simulink model "VMC_DSPLib_Solution_Stage3"  (R2025a)
settings: Solver=VariableStepAuto  StartTime=0.0  StopTime=5000  RelTol=1e-3
PreLoadFcn:
  | CreateFilter;
InitFcn:
  | CreateFilter;
undefined symbols (not defined in the file or in its folder): cfi, hb1, hb2, hb3, i, L, None, Shift1, Shift2, Shift3, ShiftCF, vsva2197, xcvc1902
libraries: aieDSP x4, dspmlti4 x3, aieBasic x1, dspsrcs4 x1, aieUtilities x1, vmcUtilities x1
settings Model: Creator=robg  LastModifiedBy=robg
settings ModelReferenceCC: EnableRefExpFcnMdlSchedulingChecks=on
settings RTWCC: GPUComputeCapability=3.5

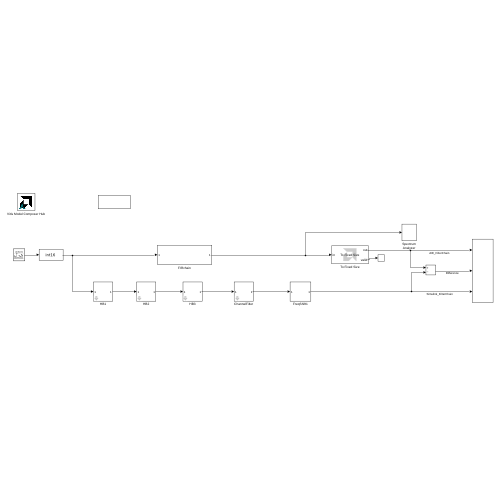
[thumbnail: Simulink's stored preview of the top-level diagram]
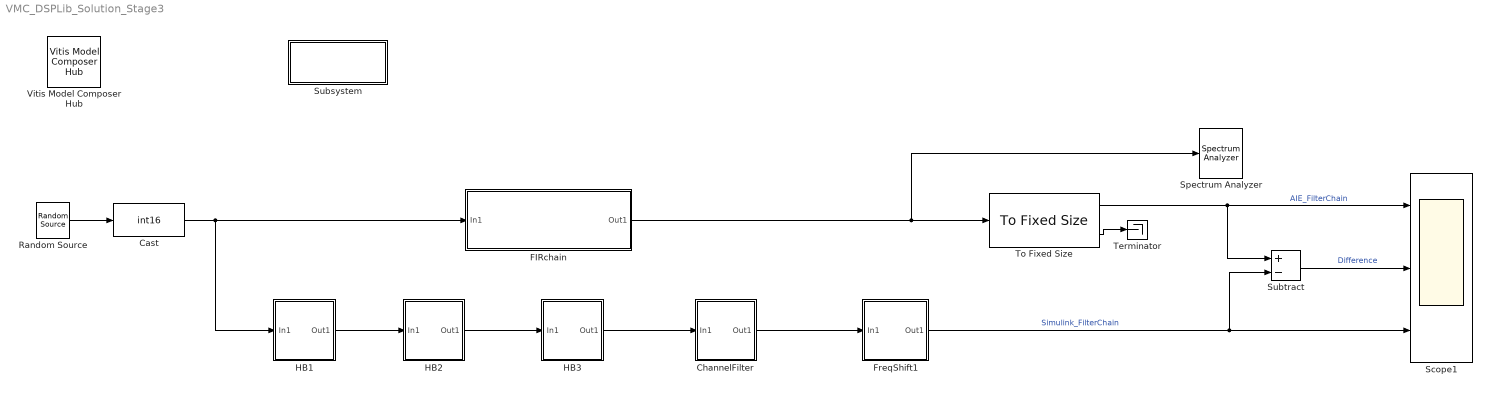
== system VMC_DSPLib_Solution_Stage3 ==
  Cast : DataTypeConversion  OutDataTypeStr=int16  SaturateOnIntegerOverflow=off  RndMeth=Floor
  ChannelFilter : Subsystem  mask{COEFFS=cfi, Shift=ShiftCF}
      mask prompts: COEFFS "Coefficients"; Shift "Final Shift"
  FIRchain : Subsystem
  FreqShift1 : Subsystem
  HB1 : Subsystem  mask{COEFFS=hb1, Shift=Shift1}
      mask prompts: COEFFS "Coefficients"; Shift "Final Shift"
  HB2 : Subsystem  mask{COEFFS=hb2, Shift=Shift2}
      mask prompts: COEFFS "Coefficients"; Shift "Final Shift"
  HB3 : Subsystem  mask{COEFFS=hb3, Shift=Shift3}
      mask prompts: COEFFS "Coefficients"; Shift "Final Shift"
  Random Source : dspsrcs4/Random Source  SrcType=Uniform  MinVal=-20000  MaxVal=20000  MeanVal=0  VarVal=1  RepMode=Specify seed  rawSeed=1  IsInherit=off  SampTime=1  SampFrame=2048  OutComplex=Complex  DataType=double  SimulateUsing=Interpreted execution
  Scope1 : Scope  NumInputPorts=3
      settings: ActiveDisplayYMinimum=-19139.5  ActiveDisplayYMaximum=19715.5
  Spectrum Analyzer : SpectrumAnalyzer  WindowPosition=[560.000000,350.000000,800.000000,500.000000,]  Visible=on  ScopeFrameLocation=window  SampleRate=0.125  Span=0.125  StartFrequency=-0.0625  StopFrequency=0.0625  AveragingMethod=Exponential  YLimits=[19.3644 90.7876]  AllowFFTLengthLessThanSamplesPerUpdate=on  DefaultConfigurationName=spbscopes.SpectrumAnalyzerBlockCfg  IsFrequencyInputMode=0  FrequencyVectorPort=0  FrequencyVectorFromPort=0  FrequencyInputRBWPort=0  FrequencyInputRBWFromPort=0
  Subsystem : Subsystem
      settings: OpenFcn=open('CreateFilter.m');
  Subtract : Sum  Inputs=+-
  Terminator : Terminator
  To Fixed Size : aieUtilities/To Fixed Size  Mode=Produce a valid output signal  OutputSize=256  CopyMethod=Buffer samples to form output  HasStatusOutput=on
  Vitis Model Composer Hub : vmcUtilities/Vitis Model Composer Hub  Tag=genX  CodeGeneration=off  SubsystemName=FIRchain  BlockHierPath=VMC_DSPLib_Solution_Stage3/FIRchain  SubsystemType=AIENode  StartColumn=1  NumberOfColumns=1  TargetDirectory=./code  exportDesign=off  analyzeDesign=on  validateDesignOnHw=off  ExportType=AI Engines  IpVendor=xilinx.com  IpLibrary=hls  IpVersion=1.0  IpHWLanguage=Verilog  AieCompilerOptions={}  AieSimulatorOptions={}  CreateTestbench=on  TestbenchStackSize=10  RunRtlSim=off  RunCSim=off  RunAieSim=on  enableSimulationTimeout=on  enableGraphIterations=on  AieSimTimeout=50000  AieGraphIterations=-1  RunAieSimProfiling=on  LaunchVitisAnalyzer=on  PlotOutput=off  RunX86Sim=off  X86SimTimeout=10  GenHwImage=off  GenLibadfXo=off  GenHwValidationCode=off  PlatformType=Not Specified  HwSystemType=Baremetal  HwValidationTarget=hw  ProjDevice=xcvc1902-vsva2197-1LHP-i-L  ProjDevicePart=xcvc1902-vsva2197-1LHP-i-L  AIEType=AIE  SamplePeriod=-1  ClockFrequency=200  DataPathParallelism=1  xilinxfamily=versalaicore  part=xcvc1902  speed=-1LHP-i-L  package=vsva2197  directory=./code  testbench=off  incr_netlist=off  synthesis_tool=Vivado  clock_wrapper=Clock Enables  dbl_ovrd=According to Block Masks  dcm_input_clock_period=10  sysclk_period=10  simulink_period=1  eval_field=0  IPInfoJsonString="{\"DUTSubsystemName\":\"FIRchain\",\"AIESubsystem\":{\"SubsystemName\":\"FIRchain\",\"TargetDirectory\":\"./code\",\"AIEArrayConfig\":\"Use entire AIE array\",\"StartColumn\":\"0\",\"NumberOfColumns\":\"1\"},\"SubsystemTag\":\"AIENode\"}"  LogFileName=/group/xcoswmktg2/robg/git/Vitis-Tutorials/Internal-Fork/AI_Engine_Development/AIE/Feature_Tutorials/10-aie-dsp-lib-model-composer/code/model_composer.log  NThreads=4  IPConfigFile=/tmp/vmctmp-2277828951318312850/VMC_DSPLib_Solution_Stage3_ipconfig.json
  wires:
  Random Source/1 -> Cast/1
  Cast/1 -> FIRchain/1(In1), HB1/1(In1)
  To Fixed Size/2 -> Terminator/1
  HB1/1(Out1) -> HB2/1(In1)
  To Fixed Size/1 -> Scope1/1, Subtract/1  "AIE_FilterChain"
  Subtract/1 -> Scope1/2  "Difference"
  HB2/1(Out1) -> HB3/1(In1)
  HB3/1(Out1) -> ChannelFilter/1(In1)
  ChannelFilter/1(Out1) -> FreqShift1/1(In1)
  FreqShift1/1(Out1) -> Scope1/3, Subtract/2  "Simulink_FilterChain"
  FIRchain/1(Out1) -> To Fixed Size/1, Spectrum Analyzer/1

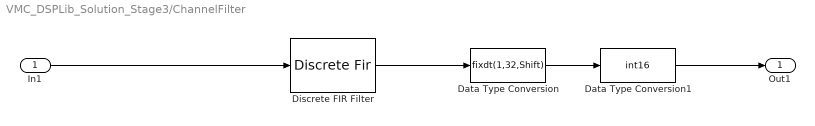
== system VMC_DSPLib_Solution_Stage3/ChannelFilter ==
  In1 : Inport
  Data Type Conversion : DataTypeConversion  OutDataTypeStr=fixdt(1,32,Shift)  ConvertRealWorld=Stored Integer (SI)  SaturateOnIntegerOverflow=off  RndMeth=Floor
  Data Type Conversion1 : DataTypeConversion  OutDataTypeStr=int16  RndMeth=Floor
  Discrete FIR Filter : DiscreteFir  Coefficients=COEFFS  InputProcessing=Columns as channels (frame based)
  Out1 : Outport
  wires:
  Data Type Conversion/1 -> Data Type Conversion1/1
  In1/1 -> Discrete FIR Filter/1
  Discrete FIR Filter/1 -> Data Type Conversion/1
  Data Type Conversion1/1 -> Out1/1

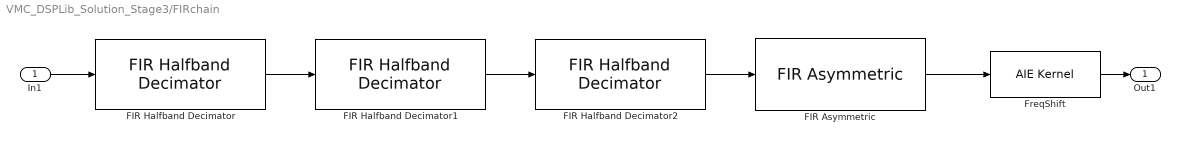
== system VMC_DSPLib_Solution_Stage3/FIRchain ==
  In1 : Inport
  FIR Asymmetric : aieDSP/FIR Asymmetric  data_type=cint16  coef_type=int16  use_coeff_reload=off  num_outputs=off  coeff=cfi  fir_length=32  input_window_size=256  shift_val=ShiftCF  rnd_mode=Floor  sat_mode=0-None  casc_length=1  AIE_VARIANT=1  TP_API=0  dual_ip=0  ssr=1  blockJsonConstraints=[]  blockJsonConstraintsInternal=[]  spec=vmc_fir_sr_asym.json  SerializedMaskParamNames=[]  SerializedMaskParamValues=[]  SerializedMaskParamVisibilities=[]  block_type=FIR Asymmetric  SerializedMaskParamDataypes=typename|typename|uint|uint|coef_type|uint|uint|uint|uint|uint|uint|uint|uint|uint|uint  SerializedMaskParamEnumStrArr=0|0|0|0|0|0|0|0|Floor,Ceiling,Round to positive infinity,Round to negative infinity,Round symmetrical to infinity,Round symmetrical to zero,Round convergent to even,Round convergent to odd|0-None,1-Asymmetric,3-Symmetric|0|0|0|0|0  SerializedMaskParamEnumValArr=0|0|0|0|0|0|0|0|0,1,2,3,4,5,6,7|0,1,3|0|0|0|0|0  SerializedMaskParamVectorArr=0|0|0|0|1|0|0|0|0|0|0|0|0|0|0  SerializedMaskParamKeys=TT_DATA|TT_COEFF|TP_USE_COEFF_RELOAD|TP_NUM_OUTPUTS|coeff|TP_FIR_LEN|TP_INPUT_WINDOW_VSIZE|TP_SHIFT|TP_RND|TP_SAT|TP_CASC_LEN|AIE_VARIANT|TP_API|TP_DUAL_IP|TP_SSR
  FIR Halfband Decimator : aieDSP/FIR Halfband Decimator  data_type=cint16  coef_type=int16  use_coeff_reload=off  dual_ip=off  num_outputs=off  coeff=hb1_aie  fir_length=31  input_window_size=2048  shift_val=Shift1  rnd_mode=Floor  sat_mode=0-None  deci_poly=1  casc_length=2  AIE_VARIANT=1  TP_API=0  ssr=1  blockJsonConstraints=[]  blockJsonConstraintsInternal=[]  spec=vmc_fir_decimate_hb.json  SerializedMaskParamNames=[]  SerializedMaskParamValues=[]  SerializedMaskParamVisibilities=[]  block_type=FIR Halfband Decimator  SerializedMaskParamDataypes=typename|typename|uint|uint|uint|coef_type|uint|uint|uint|uint|uint|uint|uint|uint|uint|uint  SerializedMaskParamEnumStrArr=0|0|0|0|0|0|0|0|0|Floor,Ceiling,Round to positive infinity,Round to negative infinity,Round symmetrical to infinity,Round symmetrical to zero,Round convergent to even,Round convergent to odd|0-None,1-Asymmetric,3-Symmetric|0|0|0|0|0  SerializedMaskParamEnumValArr=0|0|0|0|0|0|0|0|0|0,1,2,3,4,5,6,7|0,1,3|0|0|0|0|0  SerializedMaskParamVectorArr=0|0|0|0|0|1|0|0|0|0|0|0|0|0|0|0  SerializedMaskParamKeys=TT_DATA|TT_COEFF|TP_USE_COEFF_RELOAD|TP_DUAL_IP|TP_NUM_OUTPUTS|coeff|TP_FIR_LEN|TP_INPUT_WINDOW_VSIZE|TP_SHIFT|TP_RND|TP_SAT|TP_PARA_DECI_POLY|TP_CASC_LEN|AIE_VARIANT|TP_API|TP_SSR
  FIR Halfband Decimator1 : aieDSP/FIR Halfband Decimator  data_type=cint16  coef_type=int16  use_coeff_reload=off  dual_ip=off  num_outputs=off  coeff=hb2_aie  fir_length=31  input_window_size=1024  shift_val=Shift2  rnd_mode=Floor  sat_mode=0-None  deci_poly=1  casc_length=2  AIE_VARIANT=1  TP_API=0  ssr=1  blockJsonConstraints=[]  blockJsonConstraintsInternal=[]  spec=vmc_fir_decimate_hb.json  SerializedMaskParamNames=[]  SerializedMaskParamValues=[]  SerializedMaskParamVisibilities=[]  block_type=FIR Halfband Decimator  SerializedMaskParamDataypes=typename|typename|uint|uint|uint|coef_type|uint|uint|uint|uint|uint|uint|uint|uint|uint|uint  SerializedMaskParamEnumStrArr=0|0|0|0|0|0|0|0|0|Floor,Ceiling,Round to positive infinity,Round to negative infinity,Round symmetrical to infinity,Round symmetrical to zero,Round convergent to even,Round convergent to odd|0-None,1-Asymmetric,3-Symmetric|0|0|0|0|0  SerializedMaskParamEnumValArr=0|0|0|0|0|0|0|0|0|0,1,2,3,4,5,6,7|0,1,3|0|0|0|0|0  SerializedMaskParamVectorArr=0|0|0|0|0|1|0|0|0|0|0|0|0|0|0|0  SerializedMaskParamKeys=TT_DATA|TT_COEFF|TP_USE_COEFF_RELOAD|TP_DUAL_IP|TP_NUM_OUTPUTS|coeff|TP_FIR_LEN|TP_INPUT_WINDOW_VSIZE|TP_SHIFT|TP_RND|TP_SAT|TP_PARA_DECI_POLY|TP_CASC_LEN|AIE_VARIANT|TP_API|TP_SSR
  FIR Halfband Decimator2 : aieDSP/FIR Halfband Decimator  data_type=cint16  coef_type=int16  use_coeff_reload=off  dual_ip=off  num_outputs=off  coeff=hb3_aie  fir_length=31  input_window_size=512  shift_val=Shift3  rnd_mode=Floor  sat_mode=0-None  deci_poly=1  casc_length=2  AIE_VARIANT=1  TP_API=0  ssr=1  blockJsonConstraints=[]  blockJsonConstraintsInternal=[]  spec=vmc_fir_decimate_hb.json  SerializedMaskParamNames=[]  SerializedMaskParamValues=[]  SerializedMaskParamVisibilities=[]  block_type=FIR Halfband Decimator  SerializedMaskParamDataypes=typename|typename|uint|uint|uint|coef_type|uint|uint|uint|uint|uint|uint|uint|uint|uint|uint  SerializedMaskParamEnumStrArr=0|0|0|0|0|0|0|0|0|Floor,Ceiling,Round to positive infinity,Round to negative infinity,Round symmetrical to infinity,Round symmetrical to zero,Round convergent to even,Round convergent to odd|0-None,1-Asymmetric,3-Symmetric|0|0|0|0|0  SerializedMaskParamEnumValArr=0|0|0|0|0|0|0|0|0|0,1,2,3,4,5,6,7|0,1,3|0|0|0|0|0  SerializedMaskParamVectorArr=0|0|0|0|0|1|0|0|0|0|0|0|0|0|0|0  SerializedMaskParamKeys=TT_DATA|TT_COEFF|TP_USE_COEFF_RELOAD|TP_DUAL_IP|TP_NUM_OUTPUTS|coeff|TP_FIR_LEN|TP_INPUT_WINDOW_VSIZE|TP_SHIFT|TP_RND|TP_SAT|TP_PARA_DECI_POLY|TP_CASC_LEN|AIE_VARIANT|TP_API|TP_SSR
  FreqShift : aieBasic/AIE Kernel  KernelAllAttrs=|  PortNames={'in'; 'out'}  PortSerializedTypes={'{Q2{R{Tadf::input_buffer{1{t{Scint16}}}}}}'; '{Q2{R{Tadf::output_buffer{1{t{Scint16}}}}}}'}  PortWindowSizes={2.560000000000000000e+02, 2.560000000000000000e+02}  PortWindowMargins={0.000000000000000000e+00, 0.000000000000000000e+00}  PortSynchronicities={'sync', 'sync'}  PortSignalSizes={0.000000000000000000e+00; 0.000000000000000000e+00}  FunctionTemplateSpecKind=implicit  FunctionTemplateParamNames={'FRAME_LENGTH'}  FunctionTemplateParamKinds={'nontype'}  FunctionTemplateParamTypes={'int'}  FunctionTemplateParamValues={'256'}  FunctionIndex=1  FunctionTabVisible=on  FunctionTemplateParamsVisible=on  FunctionDeclTypeOptions=|  FunctionDecl=|  FunctionTemplateParams={ 'FRAME_LENGTH', 'int', '256' }  FunctionTemplateParamsEnables={'off', 'off', 'on'}  PortAttrs={ 'input', 'in', 'adf::input_buffer< cint16 > & restrict', '256', '0', 'sync', ''; 'output', 'out', 'adf::output_buffer< cint16 > & restrict', '256', '', 'sync', '' }  PortAttrsEnables={'off', 'off', 'off', 'on', 'off', 'off', 'off';'off', 'off', 'off', 'on', 'off', 'off', 'off'}  SampleTime=-1  KernelHeaderFile=aiecode_src/FreqShift.h  KernelFunction=FreqShift  KernelSourceFile=aiecode_src/FreqShift.cpp  KernelSearchPaths={}  PreProcOptions={}  blockJsonConstraints=[]
      KernelAllAttrs=|
      | s[12;12;9;9;19;14;21;23;21;23;24;21;15;17;12;24;26;26;26;27;28;9;21;23;23;23;24;25;14;19;19;29]@FunctionNameDeclFileNamePortNamesPortTypesPortSerializedTypesPortDirectionsPortWindowSizeEnablesPortWindowMarginEnablesPortBufferSizeEnablesPortBufferMarginEnablesPortSynchronicityEnablesPortSignalSizeEnablesPortBufferSizesPortBufferMarginsFunctionDeclFunctionTemplateSpecKindFunctionTemplateParamNamesFunctionTemplateParamKindsFunctionTemplateParamTypesFunctionTemplateParamValuesFunctionTemplateParamEnablesClassDeclClassTemplateSpecKindClassTemplateParamNamesClassTemplateParamKindsClassTemplateParamTypesClassTemplateParamValuesClassTemplateParamEnablesClassCtorDeclsClassCtorParamNamesClassCtorParamTypesClassCtorParamSerializedTypes[1 1]@C[32 1]@t9@FreqShiftt29@../../aiecode_src/FreqShift.hC[2 1]@t2@int3@outC[2 1]@t38@adf::input_buffer< cint16 > & restrictt39@adf::output_buffer< cint16 > & restrictC[2 1]@t42@{Q2{R{Tadf::input_buffer{1{t{Scint16}}}}}}t43@{Q2{R{Tadf::output_buffer{1{t{Scint16}}}}}}C[2 1]@t5@inputt6@outputC[2 1]@l1@l1@C[2 1]@l1@l0@C[2 1]@l1@l1@C[2 1]@l0@l0@C[2 1]@l1@l1@C[2 1]@l0@l0@C[2 1]@nnC[2 1]@nnt133@template < int FRAME_LENGTH > 
      | void FreqShift(adf::input_buffer< cint16 > & restrict in, adf::output_buffer< cint16 > & restrict out)t8@implicitC[1 1]@t12@FRAME_LENGTHC[1 1]@t7@nontypeC[1 1]@t3@intC[1 1]@nC[1 1]@l1@nne[0 1]@e[0 1]@e[0 1]@e[0 1]@e[0 1]@e[0 1]@e[0 1]@e[0 1]@e[0 1]@
      FunctionDeclTypeOptions=|
      | C[1 1]@t135@template < int FRAME_LENGTH > 
      | void FreqShift(adf::input_buffer< cint16 > && restrict in, adf::output_buffer< cint16 > && restrict out)
      FunctionDecl=|
      | template < int FRAME_LENGTH > 
      | void FreqShift(adf::input_buffer< cint16 > && restrict in, adf::output_buffer< cint16 > && restrict out)
  Out1 : Outport
  wires:
  FIR Halfband Decimator2/1 -> FIR Asymmetric/1
  FIR Halfband Decimator/1 -> FIR Halfband Decimator1/1
  FIR Halfband Decimator1/1 -> FIR Halfband Decimator2/1
  FIR Asymmetric/1 -> FreqShift/1
  FreqShift/1 -> Out1/1
  In1/1 -> FIR Halfband Decimator/1

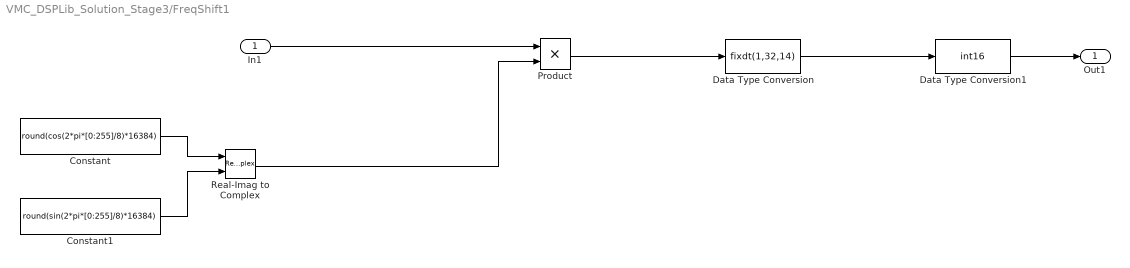
== system VMC_DSPLib_Solution_Stage3/FreqShift1 ==
  In1 : Inport
  Constant : Constant  Value=round(cos(2*pi*[0:255]/8)*16384)  SampleTime=2048
  Constant1 : Constant  Value=round(sin(2*pi*[0:255]/8)*16384)  SampleTime=2048
  Data Type Conversion : DataTypeConversion  OutDataTypeStr=fixdt(1,32,14)  ConvertRealWorld=Stored Integer (SI)  SaturateOnIntegerOverflow=off  RndMeth=Floor
  Data Type Conversion1 : DataTypeConversion  OutDataTypeStr=int16  RndMeth=Floor
  Product : Product
  Real-Imag to Complex : RealImagToComplex
  Out1 : Outport
  wires:
  In1/1 -> Product/1
  Product/1 -> Data Type Conversion/1
  Real-Imag to Complex/1 -> Product/2
  Data Type Conversion1/1 -> Out1/1
  Constant/1 -> Real-Imag to Complex/1
  Constant1/1 -> Real-Imag to Complex/2
  Data Type Conversion/1 -> Data Type Conversion1/1

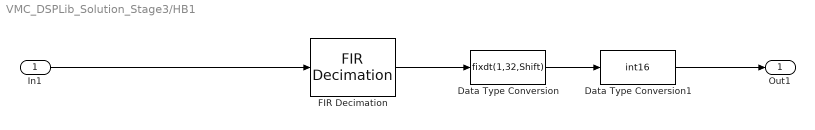
== system VMC_DSPLib_Solution_Stage3/HB1 ==
  In1 : Inport
  Data Type Conversion : DataTypeConversion  OutDataTypeStr=fixdt(1,32,Shift)  ConvertRealWorld=Stored Integer (SI)  SaturateOnIntegerOverflow=off  RndMeth=Floor
  Data Type Conversion1 : DataTypeConversion  OutDataTypeStr=int16  RndMeth=Floor
  FIR Decimation : dspmlti4/FIR Decimation  FilterSource=Dialog parameters  h=COEFFS  D=2  filtStruct=Direct form  FilterObject=FDECIM  InputProcessing=Columns as channels (frame based)  framing=Enforce single-rate processing  AllowArbitraryInputLength=off  inputOffset=0  outputBufInitCond=0  roundingMode=Floor  overflowMode=off  firstCoeffDataTypeStr=Inherit: Same word length as input  firstCoeffMin=[]  firstCoeffMax=[]  firstCoeffLastDataTypeStr=Inherit: Same word length as input  outputDataTypeStr=Inherit: Same as accumulator  outputMin=[]  outputMax=[]  outputLastDataTypeStr=Inherit: Same as accumulator
  Out1 : Outport
  wires:
  Data Type Conversion1/1 -> Out1/1
  FIR Decimation/1 -> Data Type Conversion/1
  In1/1 -> FIR Decimation/1
  Data Type Conversion/1 -> Data Type Conversion1/1

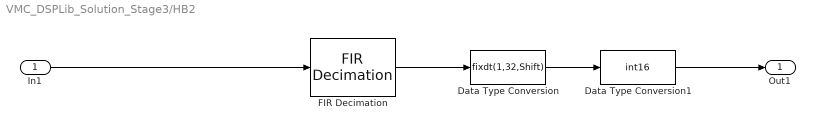
== system VMC_DSPLib_Solution_Stage3/HB2 ==
  In1 : Inport
  Data Type Conversion : DataTypeConversion  OutDataTypeStr=fixdt(1,32,Shift)  ConvertRealWorld=Stored Integer (SI)  SaturateOnIntegerOverflow=off  RndMeth=Floor
  Data Type Conversion1 : DataTypeConversion  OutDataTypeStr=int16  RndMeth=Floor
  FIR Decimation : dspmlti4/FIR Decimation  FilterSource=Dialog parameters  h=COEFFS  D=2  filtStruct=Direct form  FilterObject=FDECIM  InputProcessing=Columns as channels (frame based)  framing=Enforce single-rate processing  AllowArbitraryInputLength=off  inputOffset=0  outputBufInitCond=0  roundingMode=Floor  overflowMode=off  firstCoeffDataTypeStr=Inherit: Same word length as input  firstCoeffMin=[]  firstCoeffMax=[]  firstCoeffLastDataTypeStr=Inherit: Same word length as input  outputDataTypeStr=Inherit: Same as accumulator  outputMin=[]  outputMax=[]  outputLastDataTypeStr=Inherit: Same as accumulator
  Out1 : Outport
  wires:
  Data Type Conversion/1 -> Data Type Conversion1/1
  In1/1 -> FIR Decimation/1
  FIR Decimation/1 -> Data Type Conversion/1
  Data Type Conversion1/1 -> Out1/1

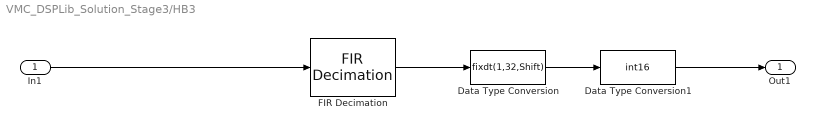
== system VMC_DSPLib_Solution_Stage3/HB3 ==
  In1 : Inport
  Data Type Conversion : DataTypeConversion  OutDataTypeStr=fixdt(1,32,Shift)  ConvertRealWorld=Stored Integer (SI)  SaturateOnIntegerOverflow=off  RndMeth=Floor
  Data Type Conversion1 : DataTypeConversion  OutDataTypeStr=int16  RndMeth=Floor
  FIR Decimation : dspmlti4/FIR Decimation  FilterSource=Dialog parameters  h=COEFFS  D=2  filtStruct=Direct form  FilterObject=FDECIM  InputProcessing=Columns as channels (frame based)  framing=Enforce single-rate processing  AllowArbitraryInputLength=off  inputOffset=0  outputBufInitCond=0  roundingMode=Floor  overflowMode=off  firstCoeffDataTypeStr=Inherit: Same word length as input  firstCoeffMin=[]  firstCoeffMax=[]  firstCoeffLastDataTypeStr=Inherit: Same word length as input  outputDataTypeStr=Inherit: Same as accumulator  outputMin=[]  outputMax=[]  outputLastDataTypeStr=Inherit: Same as accumulator
  Out1 : Outport
  wires:
  Data Type Conversion1/1 -> Out1/1
  FIR Decimation/1 -> Data Type Conversion/1
  In1/1 -> FIR Decimation/1
  Data Type Conversion/1 -> Data Type Conversion1/1

== system VMC_DSPLib_Solution_Stage3/Subsystem ==
